simulink model "Project_5_s"  (Simulink 8.4)
settings: Solver=ode5  StartTime=0.0  StopTime=10.0  FixedStep=0.01  RelTol=1e-3
values from neighbouring files (symbols this model uses):
  alpha_0 = alpha_0_d*d2r    (= 0.0630114736318)    [Project_5_m.m]
  b = 30    [Project_5_m.m]
  beta_0 = beta_0_d*d2r    (= 0)    [Project_5_m.m]
  c_D_0 = 0.01192128    [Project_5_m.m]
  c_D_alpha = c_D_alpha_d*pd2pr    (= 0.315162883663)    [Project_5_m.m]
  c_D_alphadot = c_D_alphadot_d*pd2pr    (= 0)    [Project_5_m.m]
  c_D_de = c_D_de_d*pd2pr    (= -0.0336696929435)    [Project_5_m.m]
  c_D_df = c_d_df_d*pd2pr    (= 0.0781428488889)    [Project_5_m.m]
  c_D_q = c_D_q_d*pd2pr    (= 0.180514364061)    [Project_5_m.m]
  c_L_0 = 0.004608463    [Project_5_m.m]
  c_l_0 = 0.0    (= 0)    [Project_5_m.m]
  c_L_alpha = c_L_alpha_d*pd2pr    (= 4.5530377669)    [Project_5_m.m]
  c_L_alphadot = c_L_alphadot_d*pd2pr    (= 0)    [Project_5_m.m]
  c_l_beta = c_l_beta_d*pd2pr    (= -0.0995502709884)    [Project_5_m.m]
  c_l_da = c_l_da_d*pd2pr    (= -0.122603800833)    [Project_5_m.m]
  c_L_de = c_L_de_d*pd2pr    (= 0.698939755124)    [Project_5_m.m]
  c_L_df = c_L_df_d*pd2pr    (= 0.827288030811)    [Project_5_m.m]
  c_l_dr = c_l_dr_d*pd2pr    (= 0.0274458815981)    [Project_5_m.m]
  c_l_p = c_l_p_d*pd2pr    (= -0.423611762168)    [Project_5_m.m]
  c_L_q = c_L_q_d*pd2pr    (= 2.91335287837)    [Project_5_m.m]
  c_l_r = c_l_r_d*pd2pr    (= 0.0040095128137)    [Project_5_m.m]
  c_m_0 = -0.02092347    [Project_5_m.m]
  c_m_alpha = c_m_alpha_d*pd2pr    (= -0.239914617555)    [Project_5_m.m]
  c_m_alphadot = c_m_alphadot_d*pd2pr    (= 0)    [Project_5_m.m]
  c_m_de = c_m_de_d*pd2pr    (= -0.663296050689)    [Project_5_m.m]
  c_m_df = c_m_df_d*pd2pr    (= 0.0332441571891)    [Project_5_m.m]
  c_m_q = c_m_q_d*pd2pr    (= -6.3404082567)    [Project_5_m.m]
  c_n_0 = 0.0    (= 0)    [Project_5_m.m]
  c_n_beta = c_n_beta_d*pd2pr    (= 0.18382262237)    [Project_5_m.m]
  c_n_da = c_n_da_d*pd2pr    (= -0.0118367923854)    [Project_5_m.m]
  c_n_dr = c_n_dr_d*pd2pr    (= -0.0830015309916)    [Project_5_m.m]
  c_n_p = c_n_p_d*pd2pr    (= -0.0247847218229)    [Project_5_m.m]
  c_n_r = c_n_r_d*pd2pr    (= -0.508089232439)    [Project_5_m.m]
  c_y_0 = 0.0    (= 0)    [Project_5_m.m]
  c_y_beta = c_y_beta_d*pd2pr    (= -1.25654801092)    [Project_5_m.m]
  c_y_da = c_y_da_d*pd2pr    (= 0.0282783319787)    [Project_5_m.m]
  c_y_dr = c_y_dr_d*pd2pr    (= 0.167904135947)    [Project_5_m.m]
  c_y_p = c_y_p_d*pd2pr    (= 0.0766543045372)    [Project_5_m.m]
  c_y_r = c_y_r_d*pd2pr    (= 0.538883995054)    [Project_5_m.m]
  cbar = 11.31    [Project_5_m.m]
  da = da_d*d2r    (= 0)    [Project_5_m.m]
  da_0 = da_0_d*d2r    (= 0)    [Project_5_m.m]
  de = de_d*d2r    (= 0)    [Project_5_m.m]
  de_0 = de_0_d*d2r    (= -0.0530238536908)    [Project_5_m.m]
  df_0 = df_0_d*d2r    (= 0.0261799387799)    [Project_5_m.m]
  dr = dr_d*d2r    (= -0.0349065850399)    [Project_5_m.m]
  dr_0 = dr_0_d*d2r    (= 0)    [Project_5_m.m]
  e1_0 = cos(psi_0/2)*cos(theta_0/2)*cos(phi_0/2)+sin(psi_0/2)*sin(theta_0/2)*sin(phi_0/2)    [Project_5_m.m]
  e2_0 = cos(psi_0/2)*cos(theta_0/2)*sin(phi_0/2)-sin(psi_0/2)*sin(theta_0/2)*cos(phi_0/2)    [Project_5_m.m]
  e3_0 = cos(psi_0/2)*sin(theta_0/2)*cos(phi_0/2)+sin(psi_0/2)*cos(theta_0/2)*sin(phi_0/2)    [Project_5_m.m]
  e4_0 = sin(psi_0/2)*cos(theta_0/2)*cos(phi_0/2)-cos(psi_0/2)*sin(theta_0/2)*sin(phi_0/2)    [Project_5_m.m]
  g = 32.17561865    [Project_5_m.m]
  i_xx = 8890.63    [Project_5_m.m]
  i_xy = 0.0    (= 0)    [Project_5_m.m]
  i_xz = 181.119    [Project_5_m.m]
  i_yy = 71973.5    [Project_5_m.m]
  i_yz = 0.0    (= 0)    [Project_5_m.m]
  i_zz = 77141.1    [Project_5_m.m]
  Iinv = inv(I)    [Project_5_m.m]
  mass = 762.8447    [Project_5_m.m]
  p_0 = p_0_d*d2r    (= 0)    [Project_5_m.m]
  phi_0 = phi_0_d*d2r    (= 0)    [Project_5_m.m]
  psi_0 = psi_0_d*d2r    (= 0)    [Project_5_m.m]
  q_0 = q_0_d*d2r    (= 0)    [Project_5_m.m]
  r2d = 180/pi    (= 57.2957795131)    [Project_5_m.m]
  r_0 = r_0_d*d2r    (= 0)    [Project_5_m.m]
  rho = 0.0014962376    [Project_5_m.m]
  S = 300    [Project_5_m.m]
  T_0 = 3146.482666    [Project_5_m.m]
  theta_0 = theta_0_d*d2r    (= 0.0630114736318)    [Project_5_m.m]
  V_t_0 = 626.81863    [Project_5_m.m]
settings Model: Creator=cmc4177  LastModifiedBy=cmc4177  BufferReuse=off
settings DataIOCC: SignalLoggingSaveFormat=Dataset
settings OptimizationCC: InlineParams=on  BufferReuse=off  ExpressionDepthLimit=128
settings DebuggingCC: UnderspecifiedInitializationDetection=Simplified  MergeDetectMultiDrivingBlocksExec=error  FcnCallInpInsideContextMsg=EnableAllAsError  StateNameClashWarn=none  InitInArrayFormatMsg=none
settings GRTTargetCC: CombineOutputUpdateFcns=on  GRTInterface=off

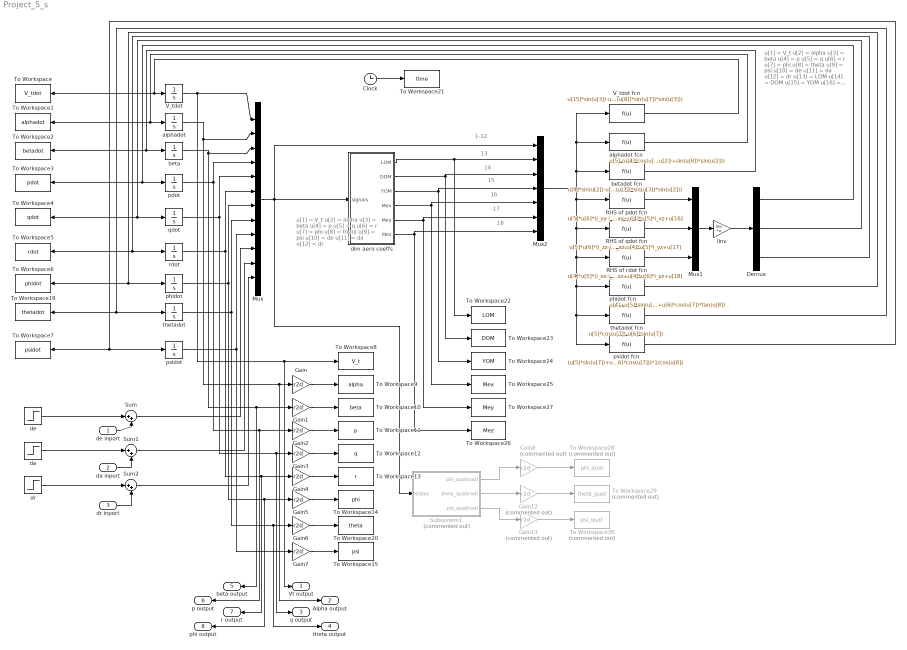
== system Project_5_s ==
  note: u[1] = V_t
      | u[2] = alpha
      | u[3] = beta
      | u[4] = p
      | u[5] = q
      | u[6] = r
      | u[7] = phi
      | u[8] = theta
      | u[9] = psi
      | u[10] = de
      | u[11] = da
      | u[12] = dr
  note: u[1] = V_t
      | u[2] = alpha
      | u[3] = beta
      | u[4] = p
      | u[5] = q
      | u[6] = r
      | u[7] = phi
      | u[8] = theta
      | u[9] = psi
      | u[10] = de
      | u[11] = da
      | u[12] = dr
      | u[13] = LOM
      | u[14] = DOM
      | u[15] = YOM
      | u[16] = Mex
      | u[17] = Mey
      | u[18] = Mez
  note: 18
  note: 17
  note: 15
  note: 14
  note: 13
  note: 1-12
  note: 16
  de inport : Inport
  da inport : Inport  Port=2
  dr inport : Inport  Port=3
  Clock : Clock
  Demux : Demux  Outputs=3
  Gain{,1..7} (8 alike) : Gain  Gain=r2d
  Gain12 : Gain  Commented=on  Gain=r2d
  Gain13 : Gain  Commented=on  Gain=r2d
  Gain8 : Gain  Commented=on  Gain=r2d
  Iinv : Gain  Gain=Iinv  Multiplication=Matrix(K*u)
  Mux : Mux  Inputs=12
  Mux1 : Mux  Inputs=3
  Mux2 : Mux  Inputs=7
  RHS of pdot fcn : Fcn  Expr=u[5]*u[6]*(i_yy-i_zz)+(u[5]*u[5]-u[6]*u[6])*i_yz-u[4]*u[6]*i_xy+u[4]*u[5]*i_xz+u[16]
  RHS of qdot fcn : Fcn  Expr=u[5]*u[6]*(i_zz-i_xx)+(u[6]*u[6]-u[4]*u[4])*i_xz-u[4]*u[5]*i_yz+u[17]
  RHS of rdot fcn : Fcn  Expr=u[4]*u[5]*(i_xx-i_yy)+(u[4]*u[4]-u[5]*u[5])*i_xy-u[5]*u[6]*i_xz+u[4]*u[6]*i_yz+u[18]
  Subsystem1 : Subsystem  Commented=on
  Sum : Sum  Inputs=|++
  Sum1 : Sum  Inputs=|++
  Sum2 : Sum  Inputs=|++
  To Workspace : ToWorkspace  VariableName=V_tdot  SampleTime=-1
  To Workspace1 : ToWorkspace  VariableName=alphadot  SampleTime=-1
  To Workspace10 : ToWorkspace  VariableName=beta  SampleTime=-1
  To Workspace11 : ToWorkspace  VariableName=p  SampleTime=-1
  To Workspace12 : ToWorkspace  VariableName=q  SampleTime=-1
  To Workspace13 : ToWorkspace  VariableName=r  SampleTime=-1
  To Workspace14 : ToWorkspace  VariableName=phi  SampleTime=-1
  To Workspace15 : ToWorkspace  VariableName=psi  SampleTime=-1
  To Workspace19 : ToWorkspace  VariableName=thetadot  SampleTime=-1
  To Workspace2 : ToWorkspace  VariableName=betadot  SampleTime=-1
  To Workspace20 : ToWorkspace  VariableName=theta  SampleTime=-1
  To Workspace21 : ToWorkspace  VariableName=time  SampleTime=-1
  To Workspace22 : ToWorkspace  VariableName=LOM  SampleTime=-1
  To Workspace23 : ToWorkspace  VariableName=DOM  SampleTime=-1
  To Workspace24 : ToWorkspace  VariableName=YOM  SampleTime=-1
  To Workspace25 : ToWorkspace  VariableName=Mex  SampleTime=-1
  To Workspace26 : ToWorkspace  VariableName=Mez  SampleTime=-1
  To Workspace27 : ToWorkspace  VariableName=Mey  SampleTime=-1
  To Workspace28 : ToWorkspace  Commented=on  VariableName=phi_quat  SampleTime=-1
  To Workspace29 : ToWorkspace  Commented=on  VariableName=theta_quat  SampleTime=-1
  To Workspace3 : ToWorkspace  VariableName=pdot  SampleTime=-1
  To Workspace30 : ToWorkspace  Commented=on  VariableName=psi_quat  SampleTime=-1
  To Workspace4 : ToWorkspace  VariableName=qdot  SampleTime=-1
  To Workspace5 : ToWorkspace  VariableName=rdot  SampleTime=-1
  To Workspace6 : ToWorkspace  VariableName=phidot  SampleTime=-1
  To Workspace7 : ToWorkspace  VariableName=psidot  SampleTime=-1
  To Workspace8 : ToWorkspace  VariableName=V_t  SampleTime=-1
  To Workspace9 : ToWorkspace  VariableName=alpha  SampleTime=-1
  V_tdot : Integrator  InitialCondition=V_t_0
  V_tdot fcn : Fcn  Expr=u[15]*sin(u[3])-u[14]*cos(u[3])+g*((cos(u[8])*cos(u[7])*sin(u[2])-sin(u[8])*cos(u[2]))*cos(u[3])+cos(u[8])*sin(u[7])*sin(u[3]))
  alphadot : Integrator  InitialCondition=alpha_0
  alphadot fcn : Fcn  Expr=u[5]-(u[4]*cos(u[2])+u[6]*sin(u[2]))*tan(u[3])-u[13]/(u[1]*cos(u[3]))+(g/(u[1]*cos(u[3])))*(cos(u[8])*cos(u[7])*cos(u[2])+sin(u[8])*sin(u[2]))
  beta : Integrator  InitialCondition=beta_0
  betadot fcn : Fcn  Expr=u[4]*sin(u[2])-u[6]*cos(u[2])+(1/u[1])*(u[15]*cos(u[3])+u[14]*sin(u[3]))+(g/u[1])*(cos(u[8])*sin(u[7])*cos(u[3])+sin(u[8])*sin(u[3])*cos(u[2])-cos(u[8])*cos(u[7])*sin(u[3])*sin(u[2]))
  da : Step  Before=da_0  After=da_0+da  SampleTime=0
  de : Step  Before=de_0  After=de_0+de  SampleTime=0
  dim aero coeffs : Subsystem
  dr : Step  Before=dr_0  After=dr_0+dr  SampleTime=0
  pdot : Integrator  InitialCondition=p_0
  phidot : Integrator  InitialCondition=phi_0
  phidot fcn : Fcn  Expr=u[4]+u[5]*sin(u[7])*tan(u[8])+u[6]*cos(u[7])*tan(u[8])
  psidot : Integrator  InitialCondition=psi_0
  psidot fcn : Fcn  Expr=(u[5]*sin(u[7])+u[6]*cos(u[7]))*1/cos(u[8])
  qdot : Integrator  InitialCondition=q_0
  rdot : Integrator  InitialCondition=r_0
  thetadot : Integrator  InitialCondition=theta_0
  thetadot fcn : Fcn  Expr=u[5]*cos(u[7])-u[6]*sin(u[7])
  Vt output : Outport
  Alpha output : Outport  Port=2
  q output : Outport  Port=3
  theta output : Outport  Port=4
  beta output : Outport  Port=5
  p output : Outport  Port=6
  r output : Outport  Port=7
  phi output : Outport  Port=8
  wires:
  V_tdot/1 -> Mux/1, Vt output/1, To Workspace8/1
  alphadot/1 -> Mux/2, Alpha output/1, Gain/1
  beta/1 -> Mux/3, beta output/1, Gain1/1
  pdot/1 -> Mux/4, p output/1, Gain2/1
  qdot/1 -> Mux/5, q output/1, Gain3/1
  psidot/1 -> Mux/9, Gain7/1
  Gain/1 -> To Workspace9/1
  Gain1/1 -> To Workspace10/1
  Gain2/1 -> To Workspace11/1
  Gain3/1 -> To Workspace12/1
  Gain4/1 -> To Workspace13/1
  Gain7/1 -> To Workspace15/1
  dr/1 -> Sum2/1
  da/1 -> Sum1/1
  de/1 -> Sum/1
  Iinv/1 -> Demux/1
  Mux1/1 -> Iinv/1
  phidot/1 -> Mux/7, phi output/1, Gain5/1
  thetadot/1 -> Mux/8, theta output/1, Gain6/1
  Gain5/1 -> To Workspace14/1
  Gain6/1 -> To Workspace20/1
  RHS of pdot fcn/1 -> Mux1/1
  RHS of qdot fcn/1 -> Mux1/2
  RHS of rdot fcn/1 -> Mux1/3
  Clock/1 -> To Workspace21/1
  V_tdot fcn/1 -> To Workspace/1, V_tdot/1
  alphadot fcn/1 -> alphadot/1, To Workspace1/1
  betadot fcn/1 -> beta/1, To Workspace2/1
  Demux/1 -> pdot/1, To Workspace3/1
  Demux/2 -> qdot/1, To Workspace4/1
  Demux/3 -> rdot/1, To Workspace5/1
  phidot fcn/1 -> phidot/1, To Workspace6/1
  thetadot fcn/1 -> thetadot/1, To Workspace19/1
  psidot fcn/1 -> To Workspace7/1, psidot/1
  Mux2/1 -> betadot fcn/1, alphadot fcn/1, V_tdot fcn/1, psidot fcn/1, thetadot fcn/1, phidot fcn/1, RHS of rdot fcn/1, RHS of qdot fcn/1, RHS of pdot fcn/1
  dim aero coeffs/1(LOM) -> Mux2/2, To Workspace22/1
  dim aero coeffs/2(DOM) -> Mux2/3, To Workspace23/1
  dim aero coeffs/3(YOM) -> Mux2/4, To Workspace24/1
  dim aero coeffs/4(Mex) -> Mux2/5, To Workspace25/1
  dim aero coeffs/6(Mez) -> Mux2/7, To Workspace26/1
  dim aero coeffs/5(Mey) -> Mux2/6, To Workspace27/1
  Gain8/1 -> To Workspace28/1
  Gain12/1 -> To Workspace29/1
  Subsystem1/1(phi_quat(rad)) -> Gain8/1
  Subsystem1/3(psi_quat(rad)) -> Gain13/1
  Subsystem1/2(theta_quat(rad)) -> Gain12/1
  Gain13/1 -> To Workspace30/1
  Mux/1 -> Mux2/1, dim aero coeffs/1(signals), Subsystem1/1(states)
  de inport/1 -> Sum/2
  da inport/1 -> Sum1/2
  dr inport/1 -> Sum2/2
  Sum2/1 -> Mux/12
  Sum1/1 -> Mux/11
  Sum/1 -> Mux/10
  rdot/1 -> Mux/6, r output/1, Gain4/1

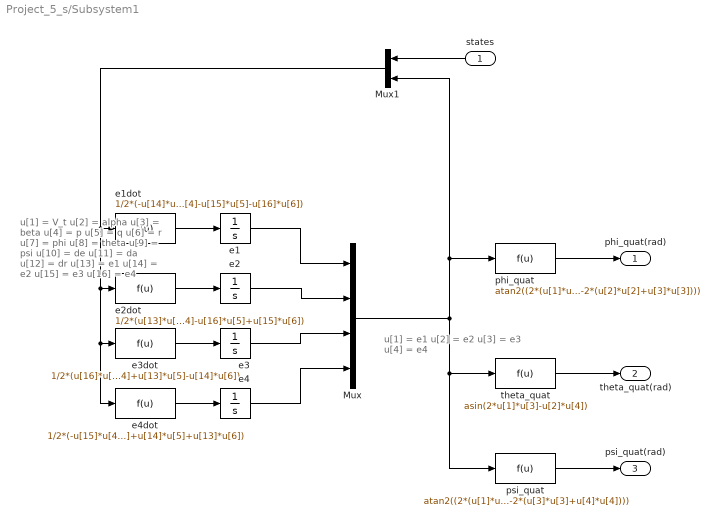
== system Project_5_s/Subsystem1 ==
  note: u[1] = e1
      | u[2] = e2
      | u[3] = e3
      | u[4] = e4
  note: u[1] = V_t
      | u[2] = alpha
      | u[3] = beta
      | u[4] = p
      | u[5] = q
      | u[6] = r
      | u[7] = phi
      | u[8] = theta
      | u[9] = psi
      | u[10] = de
      | u[11] = da
      | u[12] = dr
      | u[13] = e1
      | u[14] = e2
      | u[15] = e3
      | u[16] = e4
  states : Inport
  Mux : Mux
  Mux1 : Mux  Inputs=2
  e1 : Integrator  InitialCondition=e1_0
  e1dot : Fcn  Expr=1/2*(-u[14]*u[4]-u[15]*u[5]-u[16]*u[6])
  e2 : Integrator  InitialCondition=e2_0
  e2dot : Fcn  Expr=1/2*(u[13]*u[4]-u[16]*u[5]+u[15]*u[6])
  e3 : Integrator  InitialCondition=e3_0
  e3dot : Fcn  Expr=1/2*(u[16]*u[4]+u[13]*u[5]-u[14]*u[6])
  e4 : Integrator  InitialCondition=e4_0
  e4dot : Fcn  Expr=1/2*(-u[15]*u[4]+u[14]*u[5]+u[13]*u[6])
  phi_quat : Fcn  Expr=atan2((2*(u[1]*u[2]+u[3]*u[4])),(1-2*(u[2]*u[2]+u[3]*u[3])))
  psi_quat : Fcn  Expr=atan2((2*(u[1]*u[4]+u[2]*u[3])),(1-2*(u[3]*u[3]+u[4]*u[4])))
  theta_quat : Fcn  Expr=asin(2*u[1]*u[3]-u[2]*u[4])
  phi_quat(rad) : Outport
  theta_quat(rad) : Outport  Port=2
  psi_quat(rad) : Outport  Port=3
  wires:
  e1/1 -> Mux/1
  e2/1 -> Mux/2
  e3/1 -> Mux/3
  e4/1 -> Mux/4
  Mux/1 -> phi_quat/1, Mux1/2, theta_quat/1, psi_quat/1
  states/1 -> Mux1/1
  Mux1/1 -> e4dot/1, e3dot/1, e2dot/1, e1dot/1
  e1dot/1 -> e1/1
  e2dot/1 -> e2/1
  e3dot/1 -> e3/1
  e4dot/1 -> e4/1
  psi_quat/1 -> psi_quat(rad)/1
  theta_quat/1 -> theta_quat(rad)/1
  phi_quat/1 -> phi_quat(rad)/1

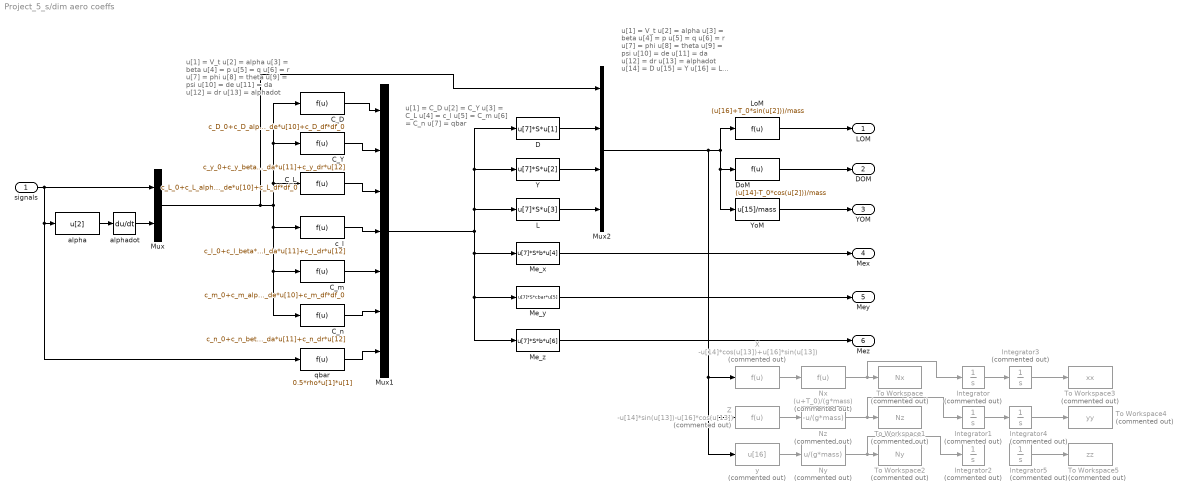
== system Project_5_s/dim aero coeffs ==
  note: u[1] = V_t
      | u[2] = alpha
      | u[3] = beta
      | u[4] = p
      | u[5] = q
      | u[6] = r
      | u[7] = phi
      | u[8] = theta
      | u[9] = psi
      | u[10] = de
      | u[11] = da
      | u[12] = dr
      | u[13] = alphadot
      | u[14] = D
      | u[15] = Y
      | u[16] = L
      | u[17] = Me_x
      | u[18] = Me_y
      | u[19] = Me_z
  note: u[1] = C_D
      | u[2] = C_Y
      | u[3] = C_L
      | u[4] = c_l
      | u[5] = C_m
      | u[6] = C_n
      | u[7] = qbar
  note: u[1] = V_t
      | u[2] = alpha
      | u[3] = beta
      | u[4] = p
      | u[5] = q
      | u[6] = r
      | u[7] = phi
      | u[8] = theta
      | u[9] = psi
      | u[10] = de
      | u[11] = da
      | u[12] = dr
      | u[13] = alphadot
  signals : Inport
  C_D : Fcn  Expr=c_D_0+c_D_alpha*u[2]+(cbar/(2*u[1]))*(c_D_q*u[5]+c_D_alphadot*u[13])+c_D_de*u[10]+c_D_df*df_0
  C_L : Fcn  Expr=c_L_0+c_L_alpha*u[2]+(cbar/(2*u[1]))*(c_L_q*u[5]+c_L_alphadot*u[13])+c_L_de*u[10]+c_L_df*df_0
  C_Y : Fcn  Expr=c_y_0+c_y_beta*u[3]+((b)/(2*u[1]))*(c_y_p*u[4]+c_y_r*u[6])+c_y_da*u[11]+c_y_dr*u[12]
  C_m : Fcn  Expr=c_m_0+c_m_alpha*u[2]+(cbar/(2*u[1]))*(c_m_q*u[5]+c_m_alphadot*u[13])+c_m_de*u[10]+c_m_df*df_0
  C_n : Fcn  Expr=c_n_0+c_n_beta*u[3]+(b/(2*u[1]))*(c_n_p*u[4]+c_n_r*u[6])+c_n_da*u[11]+c_n_dr*u[12]
  D : Fcn  Expr=u[7]*S*u[1]
  DoM : Fcn  Expr=(u[14]-T_0*cos(u[2]))/mass
  Integrator{,1..5} (6 alike) : Integrator  Commented=on
  L : Fcn  Expr=u[7]*S*u[3]
  LoM : Fcn  Expr=(u[16]+T_0*sin(u[2]))/mass
  Me_x : Fcn  Expr=u[7]*S*b*u[4]
  Me_y : Fcn  Expr=u[7]*S*cbar*u[5]
  Me_z : Fcn  Expr=u[7]*S*b*u[6]
  Mux : Mux  Inputs=2
  Mux1 : Mux  Inputs=7
  Mux2 : Mux
  Nx : Fcn  Commented=on  Expr=(u+T_0)/(g*mass)
  Ny : Fcn  Commented=on  Expr=u/(g*mass)
  Nz : Fcn  Commented=on  Expr=-u/(g*mass)
  To Workspace : ToWorkspace  Commented=on  VariableName=Nx  SaveFormat=Timeseries  SampleTime=-1
  To Workspace1 : ToWorkspace  Commented=on  VariableName=Nz  SaveFormat=Timeseries  SampleTime=-1
  To Workspace2 : ToWorkspace  Commented=on  VariableName=Ny  SaveFormat=Timeseries  SampleTime=-1
  To Workspace3 : ToWorkspace  Commented=on  VariableName=xx  SaveFormat=Timeseries  SampleTime=-1
  To Workspace4 : ToWorkspace  Commented=on  VariableName=yy  SaveFormat=Timeseries  SampleTime=-1
  To Workspace5 : ToWorkspace  Commented=on  VariableName=zz  SaveFormat=Timeseries  SampleTime=-1
  X : Fcn  Commented=on  Expr=-u[14]*cos(u[13])+u[16]*sin(u[13])
  Y : Fcn  Expr=u[7]*S*u[2]
  YoM : Fcn  Expr=u[15]/mass
  Z : Fcn  Commented=on  Expr=-u[14]*sin(u[13])-u[16]*cos(u[13])
  alpha : Fcn  Expr=u[2]
  alphadot : Derivative
  c_l : Fcn  Expr=c_l_0+c_l_beta*u[3]+(b/(2*u[1]))*(c_l_p*u[4]+c_l_r*u[6])+c_l_da*u[11]+c_l_dr*u[12]
  qbar : Fcn  Expr=0.5*rho*u[1]*u[1]
  y : Fcn  Commented=on  Expr=u[16]
  LOM : Outport
  DOM : Outport  Port=2
  YOM : Outport  Port=3
  Mex : Outport  Port=4
  Mey : Outport  Port=5
  Mez : Outport  Port=6
  wires:
  alpha/1 -> alphadot/1
  signals/1 -> qbar/1, alpha/1, Mux/1
  alphadot/1 -> Mux/2
  Mux/1 -> Mux2/1, C_L/1, C_Y/1, C_D/1, C_n/1, C_m/1, c_l/1
  C_D/1 -> Mux1/1
  C_Y/1 -> Mux1/2
  C_L/1 -> Mux1/3
  c_l/1 -> Mux1/4
  C_m/1 -> Mux1/5
  C_n/1 -> Mux1/6
  qbar/1 -> Mux1/7
  Mux1/1 -> Me_z/1, Me_y/1, Me_x/1, L/1, Y/1, D/1
  D/1 -> Mux2/2
  Y/1 -> Mux2/3
  L/1 -> Mux2/4
  Mux2/1 -> y/1, Z/1, X/1, YoM/1, DoM/1, LoM/1
  Me_x/1 -> Mex/1
  Me_y/1 -> Mey/1
  Me_z/1 -> Mez/1
  X/1 -> Nx/1
  y/1 -> Ny/1
  Z/1 -> Nz/1
  Ny/1 -> Integrator2/1, To Workspace2/1
  Nz/1 -> Integrator1/1, To Workspace1/1
  Nx/1 -> Integrator/1, To Workspace/1
  YoM/1 -> YOM/1
  DoM/1 -> DOM/1
  LoM/1 -> LOM/1
  Integrator/1 -> Integrator3/1
  Integrator1/1 -> Integrator4/1
  Integrator3/1 -> To Workspace3/1
  Integrator4/1 -> To Workspace4/1
  Integrator5/1 -> To Workspace5/1
